simulink library "radarParamConverter"  (R2021b)
settings: Solver=VariableStepAuto  StartTime=0.0  StopTime=10.0  RelTol=1e-3
settings Model: Creator=lydiazeleke  LastModifiedBy=lydiazeleke

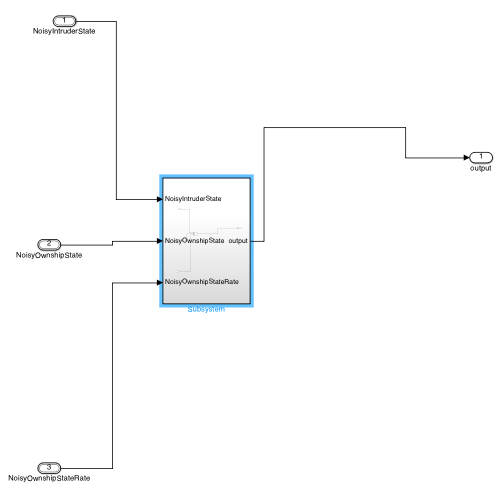
[thumbnail: Simulink's stored preview of the top-level diagram]
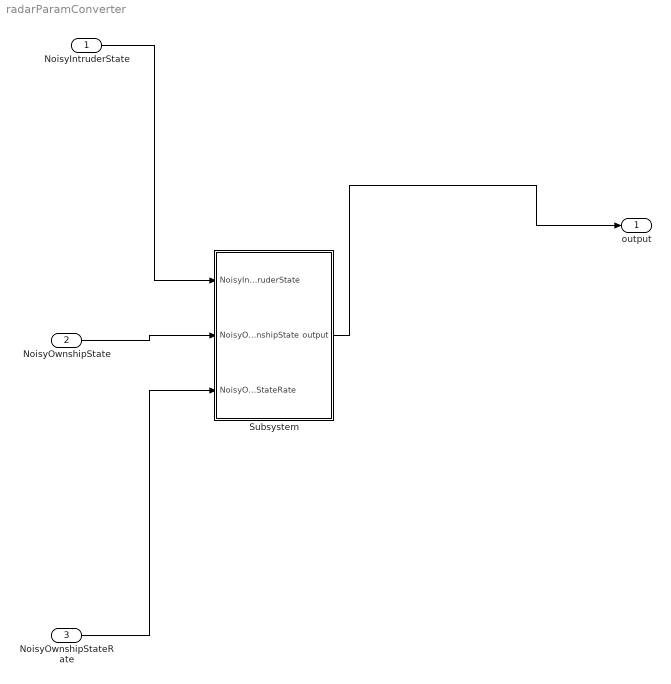
== system radarParamConverter ==
  NoisyIntruderState : Inport  OutDataTypeStr=Bus: AircraftState
  NoisyOwnshipState : Inport  Port=2  OutDataTypeStr=Bus: AircraftState
  NoisyOwnshipStateRate : Inport  Port=3  OutDataTypeStr=Bus: AircraftState
  Subsystem : Subsystem
  output : Outport  VectorParamsAs1DForOutWhenUnconnected=off
  wires:
  NoisyIntruderState/1 -> Subsystem/1(NoisyIntruderState)
  NoisyOwnshipState/1 -> Subsystem/2(NoisyOwnshipState)
  NoisyOwnshipStateRate/1 -> Subsystem/3(NoisyOwnshipStateRate)
  Subsystem/1(output) -> output/1

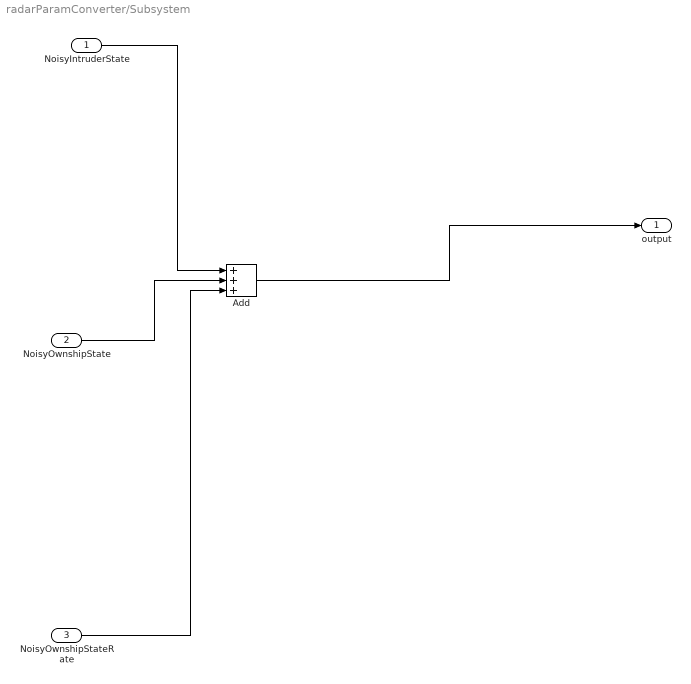
== system radarParamConverter/Subsystem ==
  NoisyIntruderState : Inport  OutDataTypeStr=Bus: AircraftState
  NoisyOwnshipState : Inport  Port=2  OutDataTypeStr=Bus: AircraftState
  NoisyOwnshipStateRate : Inport  Port=3  OutDataTypeStr=Bus: AircraftState
  Add : Sum  Inputs=+++
  output : Outport  VectorParamsAs1DForOutWhenUnconnected=off
  wires:
  NoisyIntruderState/1 -> Add/1
  Add/1 -> output/1
  NoisyOwnshipState/1 -> Add/2
  NoisyOwnshipStateRate/1 -> Add/3
